simulink model "NGV_2_6"  (R2022a)
settings: Solver=ode4  StartTime=0.0  StopTime=10.0  FixedStep=0.001  RelTol=1e-3
model workspace (MAT data in the model file):
  c = 1000
  cs = 1000
  k = 30000
  ks = 30000
  kt = 300000
  m = 500
  ms = 500
  mu = 25
settings Model: Creator=user  LastModifiedBy=ojshe
settings SolverCC: AlgebraicLoopSolver=TrustRegion
settings DebuggingCC: UnconnectedInputMsg=warning  UnconnectedOutputMsg=warning  UnconnectedLineMsg=warning  SFMachineParentedDataDiag=warning
settings RTWCC: DLArmComputeVersion=19.05

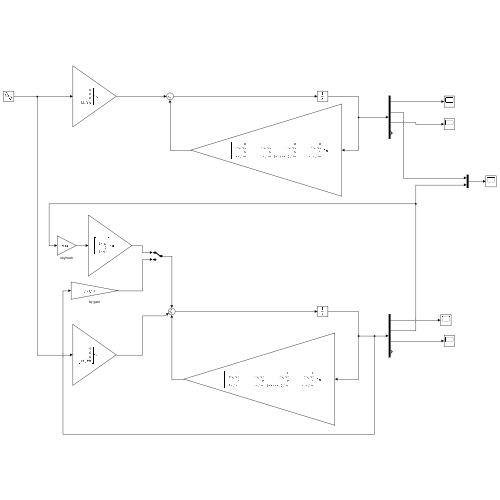
[thumbnail: Simulink's stored preview of the top-level diagram]
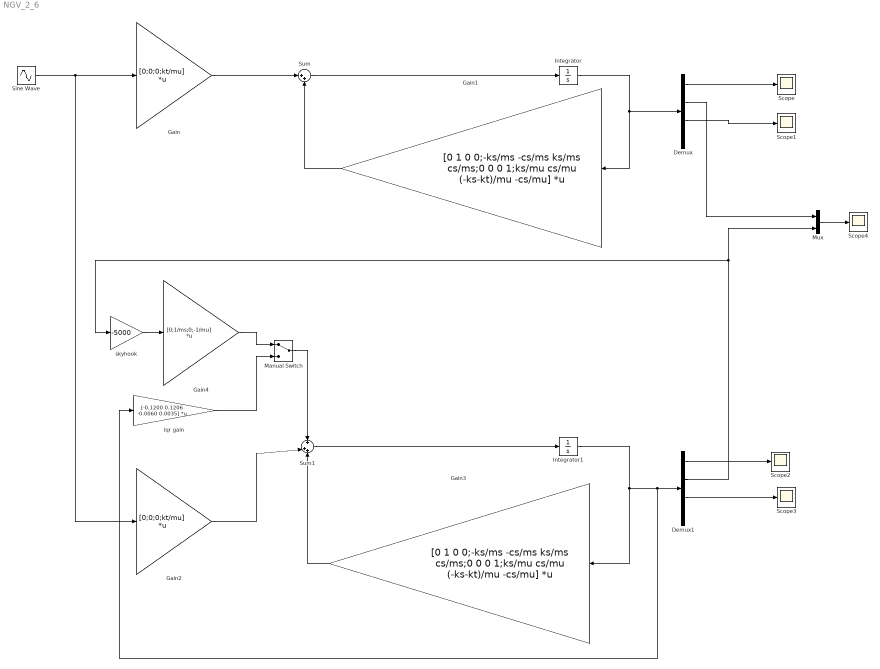
== system NGV_2_6 ==
  Demux : Demux
  Demux1 : Demux
  Gain : Gain  Gain=[0;0;0;kt/mu]  Multiplication=Matrix(K*u)
  Gain1 : Gain  Gain=[0 1 0 0;-ks/ms -cs/ms ks/ms cs/ms;0 0 0 1;ks/mu cs/mu (-ks-kt)/mu -cs/mu]  Multiplication=Matrix(K*u)
  Gain2 : Gain  Gain=[0;0;0;kt/mu]  Multiplication=Matrix(K*u)
  Gain3 : Gain  Gain=[0 1 0 0;-ks/ms -cs/ms ks/ms cs/ms;0 0 0 1;ks/mu cs/mu (-ks-kt)/mu -cs/mu]  Multiplication=Matrix(K*u)
  Gain4 : Gain  Gain=[0;1/ms;0;-1/mu]  Multiplication=Matrix(K*u)
  Integrator : Integrator
  Integrator1 : Integrator
  Manual Switch : ManualSwitch
  Mux : Mux  Inputs=2
  Scope{,1..4} (5 alike) : Scope
  Sine Wave : Sin  Amplitude=0.03  Frequency=2  SampleTime=0
  Sum : Sum  Inputs=|++
  Sum1 : Sum  Inputs=+|++
  lqr gain : Gain  Gain="[-0.1200    0.1206   -0.0060    0.0035]"  Multiplication=Matrix(K*u)
  skyhook : Gain  Gain=-5000
  wires:
  Gain/1 -> Sum/1
  Sum/1 -> Integrator/1
  Gain1/1 -> Sum/2
  Integrator/1 -> Gain1/1, Demux/1
  Demux/1 -> Scope/1
  Demux/3 -> Scope1/1
  Demux1/1 -> Scope2/1
  Sine Wave/1 -> Gain2/1, Gain/1
  Integrator1/1 -> Gain3/1, lqr gain/1, Demux1/1
  Sum1/1 -> Integrator1/1
  Gain3/1 -> Sum1/3
  Gain2/1 -> Sum1/2
  Demux1/3 -> Scope3/1
  Mux/1 -> Scope4/1
  Demux1/2 -> Mux/2, skyhook/1
  skyhook/1 -> Gain4/1
  Demux/2 -> Mux/1
  Gain4/1 -> Manual Switch/1
  lqr gain/1 -> Manual Switch/2
  Manual Switch/1 -> Sum1/1
